simulink model "simulink_problem_2_9_98"  (R2017b)
settings: Solver=VariableStepAuto  StartTime=0.0  StopTime=10.0  RelTol=1e-3
settings Model: Creator=ghost  LastModifiedBy=ghost

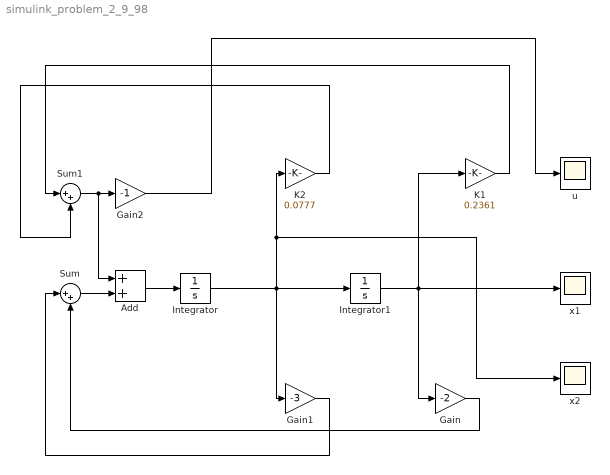
== system simulink_problem_2_9_98 ==
  Add : Sum
  Gain : Gain  Gain=-2
  Gain1 : Gain  Gain=-3
  Gain2 : Gain  Gain=-1
  Integrator : Integrator  InitialCondition=2
  Integrator1 : Integrator  InitialCondition=3
  K1 : Gain  Gain=0.2361
  K2 : Gain  Gain=0.0777
  Sum : Sum  Inputs=|++
  Sum1 : Sum  Inputs=|++
  u : Scope
  x1 : Scope
  x2 : Scope
  wires:
  Integrator/1 -> K2/1, x2/1, Gain1/1, Integrator1/1
  Integrator1/1 -> K1/1, Gain/1, x1/1
  Gain/1 -> Sum/2
  Gain1/1 -> Sum/1
  K2/1 -> Sum1/2
  K1/1 -> Sum1/1
  Sum/1 -> Add/2
  Add/1 -> Integrator/1
  Sum1/1 -> Gain2/1, Add/1
  Gain2/1 -> u/1
